simulink model "eml_karplus_strong"  (R2015a)
settings: Solver=FixedStepDiscrete  StartTime=0.0  StopTime=10  FixedStep=0.02  RelTol=1e-3
settings Model: Creator=The MathWorks, Inc.  LastModifiedBy=ktrinh
settings DataIOCC: SaveFormat=Dataset

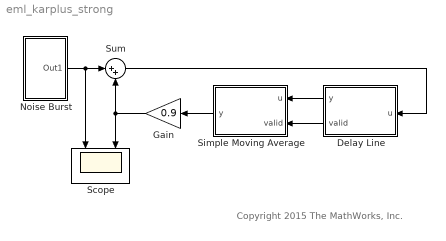
== system eml_karplus_strong ==
  note: Copyright 2015 The MathWorks, Inc.
  Delay Line : MATLAB Function  TreatAsAtomicUnit=on
      settings: PermitHierarchicalResolution=ParametersOnly
  Gain : Gain  Gain=0.9
  Noise Burst : Subsystem
  Scope : Scope  NumInputPorts=2
      settings: TimeRange=auto  MaxDataPoints=5000  SaveToWorkspace=off  SaveName=ScopeData  YMin=-1.23044~-5  YMax=1.22791~5  SampleTime=-1
  Simple Moving Average : MATLAB Function  TreatAsAtomicUnit=on
      settings: PermitHierarchicalResolution=ParametersOnly
  Sum : Sum  Inputs=|++
  wires:
  Noise Burst/1(Out1) -> Scope/1, Sum/1
  Sum/1 -> Delay Line/1(u)
  Simple Moving Average/1(y) -> Gain/1
  Gain/1 -> Sum/2, Scope/2
  Delay Line/1(y) -> Simple Moving Average/1(u)
  Delay Line/2(valid) -> Simple Moving Average/2(valid)

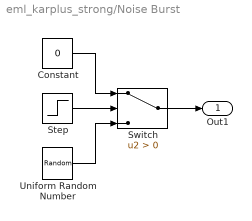
== system eml_karplus_strong/Noise Burst ==
  Constant : Constant  Value=0
  Step : Step  SampleTime=0
  Switch : Switch  Criteria=u2 > Threshold
  Uniform Random Number : UniformRandomNumber  SampleTime=0.02
  Out1 : Outport
  wires:
  Step/1 -> Switch/2
  Constant/1 -> Switch/1
  Uniform Random Number/1 -> Switch/3
  Switch/1 -> Out1/1

== matlab function eml_karplus_strong/Simple Moving Average ==
  data: u input; y output; valid input
function y = fcn(u, valid)
%#codegen

    persistent average prev_u prev_valid;
    
    if isempty(average)
        average = 0;
        prev_u = 0;
        prev_valid = false;
    end

    % Compute average
    y = average;

    % Update filter state
    if prev_valid && valid
        average = (u + prev_u) / 2;
    end
    prev_u = u;
    prev_valid = valid;
    
end

== matlab function eml_karplus_strong/Delay Line ==
  settings: updateMethod=DISCRETE
  data: u input; y output; valid output
function [y,valid] = fcn(u)
%#codegen

    persistent values counter;
    N = 48;

    if isempty(values)
        values = zeros(1, N);
        counter = 0;
    end

    % Peek at buffer head
    y = values(1);
    valid = (counter >= N);

    % Push next value
    values = [values(2:end) u];
    if counter < N
        counter = counter + 1;
    end

end
